simulink library "aerolibgravity2"  (R2020a)
settings: Solver=ode45  StartTime=0.0  StopTime=10.0  RelTol=1e-3
PostLoadFcn:
  | load_system('aerolibv1')
  | setsysloc('aerolibv1')
undefined symbols (not defined in the file or in its folder): aeroassertmsg, C, geoidgrid, ghCurrent, GM, latbp, lonbp, minYearCurrent, Newton, nMax10, nMax13, nMaxBetween, nMaxCurrent, R, Raphson, S, svCurrent, tabNMax10, tabNMax13, tabNMaxBetween
libraries: simulink x17, aerolibgravitysys x4
(part 2 of 4)

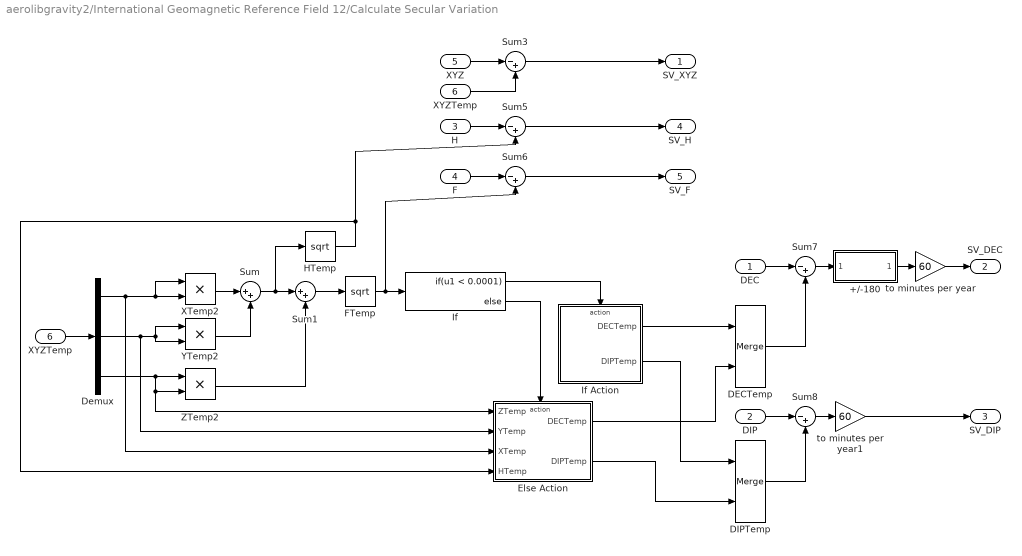
== system aerolibgravity2/International Geomagnetic Reference Field 12/Calculate Secular Variation ==
  DEC : Inport
  DIP : Inport  Port=2
  H : Inport  Port=3
  F : Inport  Port=4
  XYZ : Inport  Port=5
  XYZTemp : Inport  Port=6
  +/-180 : Subsystem
  DECTemp : Merge
  DIPTemp : Merge
  Demux : Demux  Outputs=3
  Else Action : Subsystem  TreatAsAtomicUnit=on
  FTemp : Sqrt  SaturateOnIntegerOverflow=on
  HTemp : Sqrt  SaturateOnIntegerOverflow=on
  If : If  IfExpression=u1 < 0.0001
  If Action : Subsystem  TreatAsAtomicUnit=on
  Sum : Sum  Inputs=|++
  Sum1 : Sum  Inputs=|++
  Sum{3,5..8} (5 alike) : Sum  Inputs=|-+
  XTemp2 : Product  RndMeth=Zero
  "XYZTemp " : InportShadow  Port=6
  YTemp2 : Product  RndMeth=Zero
  ZTemp2 : Product  RndMeth=Zero
  to minutes per year : Gain  Gain=60
  to minutes per year1 : Gain  Gain=60
  SV_XYZ : Outport  VectorParamsAs1DForOutWhenUnconnected=off
  SV_DEC : Outport  Port=2  VectorParamsAs1DForOutWhenUnconnected=off
  SV_DIP : Outport  Port=3  VectorParamsAs1DForOutWhenUnconnected=off
  SV_H : Outport  Port=4  VectorParamsAs1DForOutWhenUnconnected=off
  SV_F : Outport  Port=5  VectorParamsAs1DForOutWhenUnconnected=off
  wires:
  Sum3/1 -> SV_XYZ/1
  Demux/3 -> ZTemp2/1, ZTemp2/2, Else Action/1(ZTemp)
  Demux/2 -> YTemp2/2, YTemp2/1, Else Action/2(YTemp)
  Demux/1 -> XTemp2/2, XTemp2/1, Else Action/3(XTemp)
  XTemp2/1 -> Sum/1
  YTemp2/1 -> Sum/2
  Sum/1 -> Sum1/1, HTemp/1
  ZTemp2/1 -> Sum1/2
  Sum1/1 -> FTemp/1
  If/1 -> If Action/Action
  FTemp/1 -> If/1, Sum6/2
  If/2 -> Else Action/Action
  XYZ/1 -> Sum3/1
  HTemp/1 -> Else Action/4(HTemp), Sum5/2
  H/1 -> Sum5/1
  Sum5/1 -> SV_H/1
  F/1 -> Sum6/1
  Sum6/1 -> SV_F/1
  If Action/1(DECTemp) -> DECTemp/1
  Else Action/1(DECTemp) -> DECTemp/2
  DEC/1 -> Sum7/1
  DECTemp/1 -> Sum7/2
  If Action/2(DIPTemp) -> DIPTemp/1
  Else Action/2(DIPTemp) -> DIPTemp/2
  DIP/1 -> Sum8/1
  DIPTemp/1 -> Sum8/2
  Sum7/1 -> +/-180/1("DDEC ")
  Sum8/1 -> to minutes per year1/1
  to minutes per year/1 -> SV_DEC/1
  to minutes per year1/1 -> SV_DIP/1
  +/-180/1(DDEC) -> to minutes per year/1
  XYZTemp/1 -> Demux/1
  "XYZTemp "/1 -> Sum3/2

== system aerolibgravity2/International Geomagnetic Reference Field 12/Extrapolate or Interpolate ==
  dyear : Inport
  Extrapolation : Subsystem  TreatAsAtomicUnit=on
  If : If  IfExpression=u1 < 2015
  Interpolate : Subsystem  TreatAsAtomicUnit=on
  dyear1 : InportShadow
  dyear2 : InportShadow
  "gha " : Merge
  "ghb " : Merge
  "nMax " : Merge
  nMax : Outport  VectorParamsAs1DForOutWhenUnconnected=off
  gha : Outport  Port=2  VectorParamsAs1DForOutWhenUnconnected=off
  ghb : Outport  Port=3  VectorParamsAs1DForOutWhenUnconnected=off
  wires:
  If/1 -> Interpolate/Action
  If/2 -> Extrapolation/Action
  Interpolate/1(gha) -> "gha "/1
  Extrapolation/1(gha) -> "gha "/2
  Interpolate/2(ghb) -> "ghb "/1
  Extrapolation/2(ghb) -> "ghb "/2
  "gha "/1 -> gha/1
  "ghb "/1 -> ghb/1
  "nMax "/1 -> nMax/1
  Extrapolation/3(nMax) -> "nMax "/2
  Interpolate/3(nMax) -> "nMax "/1
  dyear/1 -> If/1
  dyear1/1 -> Extrapolation/1(dyear)
  dyear2/1 -> Interpolate/1(dyear)

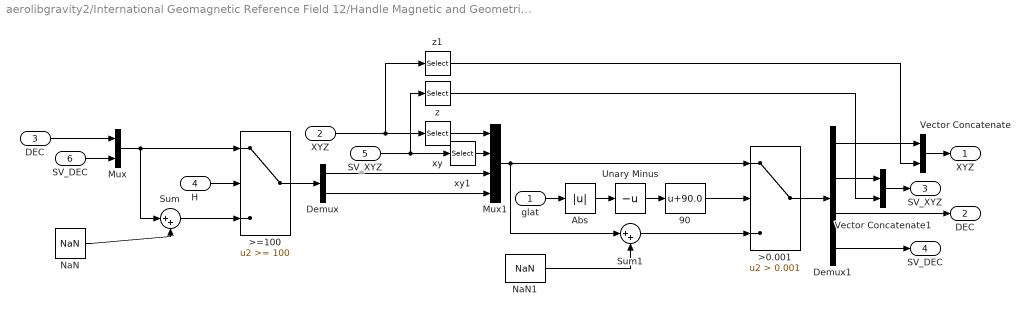
== system aerolibgravity2/International Geomagnetic Reference Field 12/Handle Magnetic and Geometric Poles ==
  glat : Inport
  "XYZ " : Inport  Port=2
  "DEC " : Inport  Port=3
  H : Inport  Port=4
  "SV_XYZ " : Inport  Port=5
  "SV_DEC " : Inport  Port=6
  90 : Bias  Bias=90.0
  >0.001 : Switch  Criteria=u2 > Threshold  Threshold=0.001
  >=100 : Switch  Threshold=100
  Abs : Abs
  Demux : Demux  Outputs=2
  Demux1 : Demux  Outputs=[2 2 1 1]
  Mux : Mux  Inputs=2
  Mux1 : Mux
  NaN : Constant  Value=NaN
  NaN1 : Constant  Value=NaN
  Sum : Sum  Inputs=|++
  Sum1 : Sum  Inputs=|++
  Unary Minus : UnaryMinus
  Vector Concatenate : Concatenate
  Vector Concatenate1 : Concatenate
  xy : Selector  InputPortWidth=3  IndexOptions=Index vector (dialog)  Indices=[1 2]  OutputSizes=1
  xy1 : Selector  InputPortWidth=3  IndexOptions=Index vector (dialog)  Indices=[1 2]  OutputSizes=1
  z : Selector  InputPortWidth=3  IndexOptions=Index vector (dialog)  Indices=3  OutputSizes=1
  z1 : Selector  InputPortWidth=3  IndexOptions=Index vector (dialog)  Indices=3  OutputSizes=1
  XYZ : Outport  Unit=nT  VectorParamsAs1DForOutWhenUnconnected=off
  DEC : Outport  Port=2  VectorParamsAs1DForOutWhenUnconnected=off
  SV_XYZ : Outport  Port=3  VectorParamsAs1DForOutWhenUnconnected=off
  SV_DEC : Outport  Port=4  VectorParamsAs1DForOutWhenUnconnected=off
  wires:
  z/1 -> Vector Concatenate1/2
  Vector Concatenate1/1 -> SV_XYZ/1
  z1/1 -> Vector Concatenate/2
  Vector Concatenate/1 -> XYZ/1
  xy1/1 -> Mux1/2
  xy/1 -> Mux1/1
  "XYZ "/1 -> z1/1, xy/1
  "SV_XYZ "/1 -> z/1, xy1/1
  H/1 -> >=100/2
  "DEC "/1 -> Mux/1
  "SV_DEC "/1 -> Mux/2
  Mux/1 -> >=100/1, Sum/1
  Sum/1 -> >=100/3
  NaN/1 -> Sum/2
  >=100/1 -> Demux/1
  Demux/1 -> Mux1/3
  Demux/2 -> Mux1/4
  glat/1 -> Abs/1
  Mux1/1 -> >0.001/1, Sum1/1
  >0.001/1 -> Demux1/1
  Demux1/1 -> Vector Concatenate/1
  Demux1/2 -> Vector Concatenate1/1
  Abs/1 -> Unary Minus/1
  Unary Minus/1 -> 90/1
  90/1 -> >0.001/2
  Demux1/3 -> DEC/1
  Demux1/4 -> SV_DEC/1
  NaN1/1 -> Sum1/2
  Sum1/1 -> >0.001/3

== system aerolibgravity2/International Geomagnetic Reference Field 12/Is decimal year within model limits ==
  u : Inport
  Assertion : Assertion  Enabled=off  AssertionFailFcn=evalin('base',callback)  StopWhenAssertionFail=off
  conjunction : Logic
  max_relop : RelationalOperator  Operator=<=  RndMeth=Nearest  InputSameDT=on
  max_val : Constant  Value=max  OutDataTypeStr=Inherit: Inherit via back propagation
  maxtype : DataTypeConversion  SaturateOnIntegerOverflow=on  RndMeth=Zero
  min_relop : RelationalOperator  Operator=<=  RndMeth=Nearest  InputSameDT=on
  min_val : Constant  Value=min  OutDataTypeStr=Inherit: Inherit via back propagation
  mintype : DataTypeConversion  SaturateOnIntegerOverflow=on  RndMeth=Zero
  out : Terminator
  wires:
  maxtype/1 -> max_relop/2
  mintype/1 -> min_relop/1
  conjunction/1 -> Assertion/1, out/1
  max_relop/1 -> conjunction/2
  min_relop/1 -> conjunction/1
  max_val/1 -> maxtype/1
  min_val/1 -> mintype/1
  u/1 -> max_relop/1, min_relop/2

== system aerolibgravity2/International Geomagnetic Reference Field 12/Length Conversion ==
  in : Inport
  Unit Conversion : UnitConversion
  out : Outport  Unit=m  VectorParamsAs1DForOutWhenUnconnected=off
  wires:
  in/1 -> Unit Conversion/1
  Unit Conversion/1 -> out/1

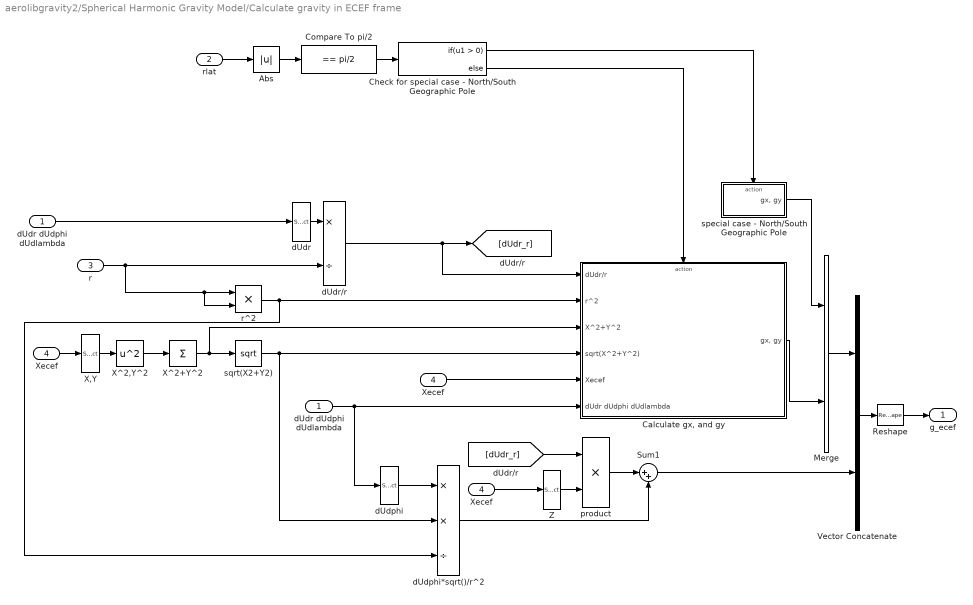
== system aerolibgravity2/Spherical Harmonic Gravity Model/Calculate gravity in ECEF frame ==
  dUdr dUdphi dUdlambda : Inport
  rlat : Inport  Port=2
  r : Inport  Port=3
  Xecef : Inport  Port=4
  " Xecef" : InportShadow  Port=4
  " Xecef " : InportShadow  Port=4
  " dUdphi " : Selector  InputPortWidth=3  IndexOptions=Index vector (dialog)  Indices=2  OutputSizes=1
  Abs : Abs
  "Calculate gx, and gy" : Subsystem
  Check for special case - North/South Geographic Pole : If
  Compare To pi/2 : simulink/Logic and Bit Operations/Compare To Constant  relop===  const=pi/2  OutDataTypeStr=uint8
  Merge : Merge
  Reshape : Reshape  OutputDimensionality=Row vector (2-D)
  Sum1 : Sum  Inputs=|++
  Vector Concatenate : Concatenate
  X,Y : Selector  InputPortWidth=3  IndexOptions=Index vector (dialog)  Indices=[1 2]  OutputSizes=1
  X^2+Y^2 : Sum  Inputs=+
  X^2,Y^2 : Math  Operator=square  SignedPower=on  SaturateOnIntegerOverflow=on
  "Z " : Selector  InputPortWidth=3  IndexOptions=Index vector (dialog)  Indices=3  OutputSizes=1
  dUdphi*sqrt()/r^2 : Product  Inputs=**/
  dUdr : Selector  InputPortWidth=3  IndexOptions=Index vector (dialog)  Indices=1  OutputSizes=1
  "dUdr dUdphi dUdlambda " : InportShadow
  dUdr/r : Product  Inputs=*/
  product : Product  RndMeth=Zero
  r^2 : Product  RndMeth=Zero
  special case - North/South Geographic Pole : Subsystem  TreatAsAtomicUnit=on
  sqrt(X2+Y2) : Sqrt  AlgorithmType=Newton-Raphson  SaturateOnIntegerOverflow=on
  g_ecef : Outport  VectorParamsAs1DForOutWhenUnconnected=off
  wires:
  rlat/1 -> Abs/1
  Merge/1 -> Vector Concatenate/1
  special case - North/South Geographic Pole/1("gx, gy") -> Merge/1
  Check for special case - North/South Geographic Pole/2 -> "Calculate gx, and gy"/Action
  "dUdr dUdphi dUdlambda "/1 -> " dUdphi "/1, "Calculate gx, and gy"/6("dUdr dUdphi dUdlambda ")
  " Xecef "/1 -> "Calculate gx, and gy"/5(" Xecef")
  Abs/1 -> Compare To pi/2/1
  Compare To pi/2/1 -> Check for special case - North/South Geographic Pole/1
  Check for special case - North/South Geographic Pole/1 -> special case - North/South Geographic Pole/Action
  Vector Concatenate/1 -> Reshape/1
  "Calculate gx, and gy"/1("gx, gy") -> Merge/2
  Sum1/1 -> Vector Concatenate/2
  " Xecef"/1 -> "Z "/1
  product/1 -> Sum1/1
  "Z "/1 -> product/2
  [dUdr_r] -> product/1
  dUdphi*sqrt()/r^2/1 -> Sum1/2
  " dUdphi "/1 -> dUdphi*sqrt()/r^2/1
  r^2/1 -> "Calculate gx, and gy"/2(r^2), dUdphi*sqrt()/r^2/3
  sqrt(X2+Y2)/1 -> dUdphi*sqrt()/r^2/2, "Calculate gx, and gy"/4(sqrt(X^2+Y^2))
  dUdr/r/1 -> "Calculate gx, and gy"/1(dUdr/r), [dUdr_r]
  X^2+Y^2/1 -> sqrt(X2+Y2)/1, "Calculate gx, and gy"/3(X^2+Y^2)
  X^2,Y^2/1 -> X^2+Y^2/1
  X,Y/1 -> X^2,Y^2/1
  dUdr/1 -> dUdr/r/1
  Reshape/1 -> g_ecef/1
  r/1 -> r^2/1, r^2/2, dUdr/r/2
  dUdr dUdphi dUdlambda/1 -> dUdr/1
  Xecef/1 -> X,Y/1

== system aerolibgravity2/Spherical Harmonic Gravity Model/Compute gravity in spherical coordinates ==
  srlon_array : Inport
  crlon_array : Inport  Port=2
  trlat : Inport  Port=3
  srphi : Inport  Port=4
  crphi : Inport  Port=5
  r : Inport  Port=6
  Compute normalized associated legendre polynomials and gravity : S-Function  FunctionName=saeroshgravity  Parameters=GM, R, C, S, int16(degree)  SFunctionDeploymentMode=off  EnableBusSupport=off
  Vector Concatenate1 : Concatenate  NumInputs=3
  dUdr dUdphi dUdlambda : Outport  VectorParamsAs1DForOutWhenUnconnected=off
  wires:
  crphi/1 -> Compute normalized associated legendre polynomials and gravity/5
  Vector Concatenate1/1 -> dUdr dUdphi dUdlambda/1
  Compute normalized associated legendre polynomials and gravity/3 -> Vector Concatenate1/3
  Compute normalized associated legendre polynomials and gravity/2 -> Vector Concatenate1/2
  Compute normalized associated legendre polynomials and gravity/1 -> Vector Concatenate1/1
  trlat/1 -> Compute normalized associated legendre polynomials and gravity/1
  srlon_array/1 -> Compute normalized associated legendre polynomials and gravity/2  "srlon"
  crlon_array/1 -> Compute normalized associated legendre polynomials and gravity/3  "crlon"
  srphi/1 -> Compute normalized associated legendre polynomials and gravity/4
  r/1 -> Compute normalized associated legendre polynomials and gravity/6

== system aerolibgravity2/Spherical Harmonic Gravity Model/Find radius, geocentric latitude, and longitude ==
  Xecef : Inport
  Divide : Product  Inputs=*/
  Dot Product : DotProduct  InputSameDT=on  OutDataTypeStr=Inherit: Inherit via internal rule
  Sum of Elements : Sum  Inputs=+
  X : Selector  InputPortWidth=3  IndexOptions=Index vector (dialog)  Indices=1  OutputSizes=1
  Y : Selector  InputPortWidth=3  IndexOptions=Index vector (dialog)  Indices=2  OutputSizes=1
  Z : Selector  InputPortWidth=3  IndexOptions=Index vector (dialog)  Indices=3  OutputSizes=1
  "r " : Sqrt  AlgorithmType=Newton-Raphson  SaturateOnIntegerOverflow=on
  "rlat " : Trigonometry  Operator=asin
  "rlon " : Trigonometry  Operator=atan2
  rlon : Outport  VectorParamsAs1DForOutWhenUnconnected=off
  rlat : Outport  Port=2  VectorParamsAs1DForOutWhenUnconnected=off
  r : Outport  Port=3  VectorParamsAs1DForOutWhenUnconnected=off
  wires:
  Y/1 -> "rlon "/1
  X/1 -> "rlon "/2
  "rlon "/1 -> rlon/1
  "rlat "/1 -> rlat/1
  Z/1 -> Divide/1
  Divide/1 -> "rlat "/1
  "r "/1 -> r/1, Divide/2
  Sum of Elements/1 -> "r "/1
  Dot Product/1 -> Sum of Elements/1
  Xecef/1 -> X/1, Y/1, Dot Product/2, Dot Product/1, Z/1

== system aerolibgravity2/Spherical Harmonic Gravity Model/Get Cosine and Sine of Latitude and Longitude ==
  rlon : Inport
  rlat : Inport  Port=2
  Constant : Constant  Value=pi/2
  Demux : Demux  Outputs=2
      settings: DisplayOption=none
  Demux1 : Demux  Outputs=2
      settings: DisplayOption=none
  Mux : Mux  Inputs=2
  Sum : Sum  Inputs=|-+
  Test for less than eps : Subsystem
  "Test for less than eps " : Subsystem
  sincos : Trigonometry  Operator=sincos
  sincos1 : Trigonometry  Operator=tan
  srlon : Outport  VectorParamsAs1DForOutWhenUnconnected=off
  crlon : Outport  Port=2  VectorParamsAs1DForOutWhenUnconnected=off
  trlat : Outport  Port=3  VectorParamsAs1DForOutWhenUnconnected=off
  srphi : Outport  Port=4  VectorParamsAs1DForOutWhenUnconnected=off
  crphi : Outport  Port=5  VectorParamsAs1DForOutWhenUnconnected=off
  wires:
  "Test for less than eps "/1(Out1) -> crphi/1
  Test for less than eps/1(Out1) -> srphi/1
  sincos1/1 -> trlat/1
  Constant/1 -> Sum/2
  Sum/1 -> Mux/2
  Mux/1 -> sincos/1
  sincos/1 -> Demux/1
  sincos/2 -> Demux1/1
  rlon/1 -> Mux/1
  rlat/1 -> Sum/1, sincos1/1
  Demux/1 -> srlon/1
  Demux1/1 -> crlon/1
  Demux/2 -> Test for less than eps/1(In1)
  Demux1/2 -> "Test for less than eps "/1(In1)

== system aerolibgravity2/Spherical Harmonic Gravity Model/sin(m_lon) & cos(m_lon) ==
  srlon : Inport
  crlon : Inport  Port=2
  For Iterator Subsystem : Subsystem  TreatAsAtomicUnit=on
  Test for less than eps : Subsystem
  "Test for less than eps " : Subsystem
  srlon_array : Outport  InitialOutput=[ zeros(1,degree+1) ]  VectorParamsAs1DForOutWhenUnconnected=off
  crlon_array : Outport  Port=2  InitialOutput=[ zeros(1,degree+1) ]  VectorParamsAs1DForOutWhenUnconnected=off
  wires:
  "Test for less than eps "/1(Out1) -> For Iterator Subsystem/2(crlon[1])
  srlon/1 -> Test for less than eps/1(In1)
  crlon/1 -> "Test for less than eps "/1(In1)
  For Iterator Subsystem/1(srlon_array) -> srlon_array/1
  For Iterator Subsystem/2(crlon_array) -> crlon_array/1
  Test for less than eps/1(Out1) -> For Iterator Subsystem/1(srlon[1])

== system aerolibgravity2/World Magnetic Model/Is time within model limits ==
  u : Inport
  Assertion : Assertion  AssertionFailFcn=evalin('base',callback)
  conjunction : Logic
  max_relop : RelationalOperator  Operator=<=  RndMeth=Nearest  InputSameDT=on
  max_val : Constant  Value=max
  maxtype : DataTypeConversion  SaturateOnIntegerOverflow=on  RndMeth=Zero
  min_relop : RelationalOperator  Operator=<=  RndMeth=Nearest  InputSameDT=on
  min_val : Constant  Value=min
  mintype : DataTypeConversion  SaturateOnIntegerOverflow=on  RndMeth=Zero
  out : Terminator
  wires:
  maxtype/1 -> max_relop/2
  mintype/1 -> min_relop/1
  conjunction/1 -> Assertion/1, out/1
  max_relop/1 -> conjunction/2
  min_relop/1 -> conjunction/1
  max_val/1 -> maxtype/1
  min_val/1 -> mintype/1
  u/1 -> max_relop/1, min_relop/2

== system aerolibgravity2/World Magnetic Model/Length Conversion ==
  in : Inport
  Unit Conversion : UnitConversion
  out : Outport  Unit=m  VectorParamsAs1DForOutWhenUnconnected=off
  wires:
  in/1 -> Unit Conversion/1
  Unit Conversion/1 -> out/1

== system aerolibgravity2/World Magnetic Model/MagField Conversion ==
  in : Inport  Unit=nT
  Unit Conversion : UnitConversion
  out : Outport  Unit=nT  VectorParamsAs1DForOutWhenUnconnected=off
  wires:
  in/1 -> Unit Conversion/1
  Unit Conversion/1 -> out/1

== system aerolibgravity2/World Magnetic Model/MagField Conversion1 ==
  in : Inport  Unit=nT
  Unit Conversion : UnitConversion
  out : Outport  Unit=nT  VectorParamsAs1DForOutWhenUnconnected=off
  wires:
  in/1 -> Unit Conversion/1
  Unit Conversion/1 -> out/1

== system aerolibgravity2/Zonal Harmonic Gravity Model/Calculate gravity in ECEF frame ==
  g_radial : Inport
  g_trans : Inport  Port=2
  r : Inport  Port=3
  Xecef : Inport  Port=4
  Divide : Product  Inputs=*/
  Mux : Mux  Inputs=3
  Reshape : Reshape  OutputDimensionality=Row vector (2-D)
  gx & gy : Subsystem
  gz : Subsystem
  g_ecef : Outport  VectorParamsAs1DForOutWhenUnconnected=off
  wires:
  Reshape/1 -> g_ecef/1
  gz/1(gz) -> Mux/3
  gx & gy/2(gy) -> Mux/2
  gx & gy/1(gx) -> Mux/1
  Mux/1 -> Reshape/1
  g_trans/1 -> gx & gy/2(g_trans), gz/3(g_trans)
  Divide/1 -> gx & gy/4(g_radial/r), gz/1(g_radial/r)
  r/1 -> gx & gy/3(r), gz/2(r), Divide/2
  g_radial/1 -> Divide/1
  Xecef/1 -> gz/4(Xecef), gx & gy/1(Xecef)

== system aerolibgravity2/Zonal Harmonic Gravity Model/Find radius and geocentric latitude ==
  Xecef : Inport
  Divide : Product  Inputs=*/
  Dot Product : DotProduct  InputSameDT=on  OutDataTypeStr=Inherit: Inherit via internal rule
  Selector : Selector  InputPortWidth=3  IndexOptions=Index vector (dialog)  Indices=3  OutputSizes=1
  Sum of Elements : Sum  Inputs=+
  "rlat " : Trigonometry  Operator=asin
  sqrt : Sqrt  AlgorithmType=Newton-Raphson  SaturateOnIntegerOverflow=on
  rlat : Outport  VectorParamsAs1DForOutWhenUnconnected=off
  r : Outport  Port=2  VectorParamsAs1DForOutWhenUnconnected=off
  wires:
  "rlat "/1 -> rlat/1
  Selector/1 -> Divide/1
  Divide/1 -> "rlat "/1
  sqrt/1 -> r/1, Divide/2
  Sum of Elements/1 -> sqrt/1
  Dot Product/1 -> Sum of Elements/1
  Xecef/1 -> Dot Product/1, Dot Product/2, Selector/1

== system aerolibgravity2/Geoid Height/Format Output/Change Units ==
  in : Inport  Unit=m
  Unit Conversion : UnitConversion
  out : Outport  Unit=m  VectorParamsAs1DForOutWhenUnconnected=off
  wires:
  in/1 -> Unit Conversion/1
  Unit Conversion/1 -> out/1

== system aerolibgravity2/Geoid Height/Format Output/Truncate ==
  In1 : Inport
  Constant1 : Constant  Value=100  OutDataTypeStr=double
  Divide : Product  Inputs=*/
  Product : Product  RndMeth=Zero
  Rounding Function : Rounding  Operator=fix
  Out1 : Outport  VectorParamsAs1DForOutWhenUnconnected=off
  wires:
  Divide/1 -> Out1/1
  In1/1 -> Product/1
  Constant1/1 -> Divide/2, Product/2
  Rounding Function/1 -> Divide/1
  Product/1 -> Rounding Function/1

== system aerolibgravity2/Geoid Height/Format Output/Truncate1 ==
  In1 : Inport
  Constant1 : Constant  Value=100  OutDataTypeStr=double
  Divide : Product  Inputs=*/
  Product : Product  RndMeth=Zero
  Rounding Function : Rounding  Operator=fix
  Out1 : Outport  VectorParamsAs1DForOutWhenUnconnected=off
  wires:
  Product/1 -> Rounding Function/1
  Rounding Function/1 -> Divide/1
  Constant1/1 -> Product/2, Divide/2
  In1/1 -> Product/1
  Divide/1 -> Out1/1

== system aerolibgravity2/Geoid Height/Wrap Latitude/If Action Subsystem ==
  Lat : Inport
  Lon : Inport  Port=2
  Action Port : ActionPort  PropagateVarSize=During execution
  Abs : Abs
  Add : Sum
  Add1 : Sum  Inputs=-+
  Add2 : Sum  Inputs=+-
  Constant1 : Constant  Value=double(90)
  Constant2 : Constant  Value=double(180)
  Divide : Product  Inputs=**
  Sign : Signum
  Lat1 : Outport  VectorParamsAs1DForOutWhenUnconnected=off
  Lon1 : Outport  Port=2  VectorParamsAs1DForOutWhenUnconnected=off
  wires:
  Lon/1 -> Add/1
  Constant2/1 -> Add/2
  Add/1 -> Lon1/1
  Divide/1 -> Lat1/1
  Abs/1 -> Add2/1
  Add2/1 -> Add1/1
  Constant1/1 -> Add2/2, Add1/2
  Sign/1 -> Divide/1
  Add1/1 -> Divide/2
  Lat/1 -> Abs/1, Sign/1

== system aerolibgravity2/Geoid Height/Wrap Latitude/If Action Subsystem1 ==
  Lat : Inport
  Lon : Inport  Port=2
  Action Port : ActionPort  PropagateVarSize=During execution
  Lat1 : Outport  VectorParamsAs1DForOutWhenUnconnected=off
  Lon1 : Outport  Port=2  VectorParamsAs1DForOutWhenUnconnected=off
  wires:
  Lat/1 -> Lat1/1
  Lon/1 -> Lon1/1

== system aerolibgravity2/Geoid Height/Wrap Latitude/Wrap Latitude 180 ==
  lat : Inport
  Constant : Constant  Value=double(360)
  Constant1 : Constant  Value=double(180)
  Math Function : Math  Operator=mod  SignedPower=on  SaturateOnIntegerOverflow=on
  Sum : Sum  Inputs=++|
  Sum1 : Sum  Inputs=-+|
  lat 180 : Outport  VectorParamsAs1DForOutWhenUnconnected=off
  wires:
  lat/1 -> Sum/2
  Sum/1 -> Math Function/1
  Constant/1 -> Math Function/2
  Math Function/1 -> Sum1/2
  Sum1/1 -> lat 180/1
  Constant1/1 -> Sum/1, Sum1/1

== system aerolibgravity2/Geoid Height/Wrap Longitude/If Action Subsystem ==
  Lon : Inport
  Action Port : ActionPort  PropagateVarSize=During execution
  Constant1 : Constant  Value=double(360)
  Math Function : Math  Operator=mod  SignedPower=on  SaturateOnIntegerOverflow=on
  Lon1 : Outport  VectorParamsAs1DForOutWhenUnconnected=off
  wires:
  Constant1/1 -> Math Function/2
  Lon/1 -> Math Function/1
  Math Function/1 -> Lon1/1

== system aerolibgravity2/Geoid Height/Wrap Longitude/If Action Subsystem1 ==
  Lon : Inport
  Action Port : ActionPort  PropagateVarSize=During execution
  Lon1 : Outport  VectorParamsAs1DForOutWhenUnconnected=off
  wires:
  Lon/1 -> Lon1/1

== system aerolibgravity2/International Geomagnetic Reference Field 12/Calculate Field/Compute magnetic vector in spherical coordinates ==
  gha : Inport
  ghb : Inport  Port=2
  r : Inport  Port=3
  clat : Inport  Port=4
  slat : Inport  Port=5
  sd : Inport  Port=6
  cd : Inport  Port=7
  crlon : Inport  Port=8
  srlon : Inport  Port=9
  nMax : Inport  Port=10
  Enable : EnablePort  PropagateVarSize=During execution
  "Calculate X, Z, XTemp and ZTemp" : Subsystem
  Compute magnetic vector in spherical coordinates : Subsystem  TreatAsAtomicUnit=on
  Constant2 : Constant  Value=0.5  OutDataTypeStr=Inherit: Inherit via back propagation
  Product3 : Product  Inputs=***  SaturateOnIntegerOverflow=on  OutDataTypeStr=Inherit: Same as first input
  aor : Product  Inputs=*/  SaturateOnIntegerOverflow=on  OutDataTypeStr=Inherit: Same as first input
  nMax+3 : Bias  Bias=3.0
  re : Constant  Value=6371.2  OutDataTypeStr=Inherit: Inherit via back propagation
  XYZ : Outport  InitialOutput=[0 0 0]  VectorParamsAs1DForOutWhenUnconnected=off
  XYZTemp : Outport  Port=2  InitialOutput=[0 0 0]  VectorParamsAs1DForOutWhenUnconnected=off
  wires:
  Product3/1 -> Compute magnetic vector in spherical coordinates/8(cntMax)
  Constant2/1 -> Product3/3
  nMax+3/1 -> Product3/2
  nMax/1 -> Product3/1, nMax+3/1
  gha/1 -> Compute magnetic vector in spherical coordinates/1(gha)
  ghb/1 -> Compute magnetic vector in spherical coordinates/2(ghb)
  re/1 -> aor/1
  aor/1 -> Compute magnetic vector in spherical coordinates/3(aor)
  Compute magnetic vector in spherical coordinates/1(XYZ) -> "Calculate X, Z, XTemp and ZTemp"/1("XYZ ")
  Compute magnetic vector in spherical coordinates/2(XYZTemp) -> "Calculate X, Z, XTemp and ZTemp"/2("XYZTemp ")
  "Calculate X, Z, XTemp and ZTemp"/1(XYZ) -> XYZ/1
  "Calculate X, Z, XTemp and ZTemp"/2(XYZTemp) -> XYZTemp/1
  r/1 -> aor/2
  clat/1 -> Compute magnetic vector in spherical coordinates/4(clat)
  slat/1 -> Compute magnetic vector in spherical coordinates/5(slat)
  crlon/1 -> Compute magnetic vector in spherical coordinates/6(crlon)
  srlon/1 -> Compute magnetic vector in spherical coordinates/7(srlon)
  sd/1 -> "Calculate X, Z, XTemp and ZTemp"/3(sd)
  cd/1 -> "Calculate X, Z, XTemp and ZTemp"/4(cd)

== system aerolibgravity2/International Geomagnetic Reference Field 12/Calculate Field/Convert from geodetic to spherical coordinates ==
  alt : Inport
  srlat : Inport  Port=2
  srlat2 : Inport  Port=3
  crlat2 : Inport  Port=4
  crlat : Inport  Port=5
  Enable : EnablePort  PropagateVarSize=During execution
  Demux : Demux
      settings: DisplayOption=none
  Demux1 : Demux
      settings: DisplayOption=none
  Demux3 : Demux  Outputs=2
      settings: DisplayOption=none
  Mux : Mux
  Selector : Selector  InputPortWidth=4  IndexOptions=Index vector (dialog)  Indices=[1 2]  OutputSizes=1
  a2 : Constant  Value=40680631.59  OutDataTypeStr=Inherit: Inherit via back propagation
  "alt " : InportShadow
  b2 : Constant  Value=40408299.98  OutDataTypeStr=Inherit: Inherit via back propagation
  calculate cd : Subsystem
  calculate clat & slat : Subsystem
  calculate d : Subsystem
  calculate r2 : Subsystem
  calculate sd : Subsystem
  r : Outport  InitialOutput=[40680631]  VectorParamsAs1DForOutWhenUnconnected=off
  clat : Outport  Port=2  InitialOutput=[0]  VectorParamsAs1DForOutWhenUnconnected=off
  slat : Outport  Port=3  InitialOutput=[1]  VectorParamsAs1DForOutWhenUnconnected=off
  sd : Outport  Port=4  InitialOutput=[0]  VectorParamsAs1DForOutWhenUnconnected=off
  cd : Outport  Port=5  InitialOutput=[0]  VectorParamsAs1DForOutWhenUnconnected=off
  wires:
  Demux/3 -> calculate d/3(srlat2)
  Selector/1 -> Demux3/1
  Demux3/2 -> calculate sd/3(b2)
  Demux3/1 -> calculate sd/2(a2)
  Mux/1 -> Demux/1, Demux1/1, Selector/1
  Demux1/3 -> calculate r2/4(srlat2)
  Demux1/2 -> calculate r2/3(b2)
  Demux1/1 -> calculate r2/2(a2)
  Demux/1 -> calculate d/1(a2)
  Demux/2 -> calculate d/2(b2)
  b2/1 -> Mux/2
  a2/1 -> Mux/1
  calculate sd/1(sd) -> calculate clat & slat/1(sd), sd/1
  crlat/1 -> calculate sd/5(crlat), calculate clat & slat/3(crlat)
  calculate cd/1(cd) -> cd/1, calculate clat & slat/4(cd)
  calculate d/2(d) -> calculate sd/1(d), calculate cd/3(d), calculate r2/7(d)
  calculate r2/1(r) -> calculate cd/2(r), calculate sd/4(r), r/1
  calculate clat & slat/2(slat) -> slat/1  "slat"
  calculate clat & slat/1(clat) -> clat/1  "clat"
  srlat/1 -> calculate sd/6(srlat), calculate clat & slat/2(srlat)
  crlat2/1 -> Mux/4
  alt/1 -> calculate r2/1(alt)
  srlat2/1 -> Mux/3
  Demux/4 -> calculate d/4(crlat2)
  Demux1/4 -> calculate r2/5(crlat2)
  calculate d/1(c2) -> calculate r2/6(c2)
  "alt "/1 -> calculate cd/1(alt)

== system aerolibgravity2/International Geomagnetic Reference Field 12/Calculate Field/Get Cosine and Sine of Latitude and Longitude ==
  lon : Inport  Unit=deg
  lat : Inport  Port=2  Unit=deg
  Enable : EnablePort  PropagateVarSize=During execution
  300 ft from North & South poles : Subsystem
  Angle Conversion : Subsystem
  Demux : Demux  Outputs=2
      settings: DisplayOption=none
  Demux1 : Demux  Outputs=2
      settings: DisplayOption=none
  Mux : Mux  Inputs=2
  Product : Product  OutDataTypeStr=Inherit: Inherit via back propagation  SaturateOnIntegerOverflow=on
  Product1 : Product  OutDataTypeStr=Inherit: Inherit via back propagation  SaturateOnIntegerOverflow=on
  sincos : Trigonometry  Operator=sincos
  srlat : Outport  InitialOutput=[0]  VectorParamsAs1DForOutWhenUnconnected=off
  srlat2 : Outport  Port=2  InitialOutput=[0]  VectorParamsAs1DForOutWhenUnconnected=off
  crlat2 : Outport  Port=3  InitialOutput=[0]  VectorParamsAs1DForOutWhenUnconnected=off
  crlat : Outport  Port=4  InitialOutput=[0]  VectorParamsAs1DForOutWhenUnconnected=off
  crlon : Outport  Port=5  InitialOutput=[1]  VectorParamsAs1DForOutWhenUnconnected=off
  srlon : Outport  Port=6  InitialOutput=[0]  VectorParamsAs1DForOutWhenUnconnected=off
  wires:
  Demux1/2 -> 300 ft from North & South poles/1("crlat ")
  Demux/2 -> Product/2, Product/1, srlat/1
  Product1/1 -> crlat2/1
  Product/1 -> srlat2/1
  Demux1/1 -> crlon/1  "crlon"
  Demux/1 -> srlon/1  "srlon"
  lat/1 -> Mux/2
  lon/1 -> Mux/1
  sincos/2 -> Demux1/1
  sincos/1 -> Demux/1
  Mux/1 -> Angle Conversion/1(in)
  Angle Conversion/1(out) -> sincos/1
  300 ft from North & South poles/1(crlat) -> Product1/2, Product1/1, crlat/1

== system aerolibgravity2/International Geomagnetic Reference Field 12/Calculate Field/Has altitude or latitude changed ==
  lat : Inport
  alt : Inport  Port=2
  Logical Operator : Logic  Operator=OR  AllPortsSameDT=off
  Relational Operator : RelationalOperator  Operator=~=  RndMeth=Nearest
  Relational Operator1 : RelationalOperator  Operator=~=  RndMeth=Nearest
  oalt : Memory  InitialCondition=-1000  InheritSampleTime=on
  olat : Memory  InitialCondition=-1000  InheritSampleTime=on
  Alt_Lat change : Outport  VectorParamsAs1DForOutWhenUnconnected=off
  wires:
  Logical Operator/1 -> Alt_Lat change/1
  lat/1 -> olat/1, Relational Operator/1
  Relational Operator1/1 -> Logical Operator/2
  Relational Operator/1 -> Logical Operator/1
  oalt/1 -> Relational Operator1/2
  olat/1 -> Relational Operator/2
  alt/1 -> oalt/1, Relational Operator1/1

== system aerolibgravity2/International Geomagnetic Reference Field 12/Calculate Field/Has longitude changed  ==
  lon : Inport
  Relational Operator : RelationalOperator  Operator=~=  RndMeth=Nearest
  olon : Memory  InitialCondition=-1000  InheritSampleTime=on
  Longitude change : Outport  VectorParamsAs1DForOutWhenUnconnected=off
  wires:
  Relational Operator/1 -> Longitude change/1
  lon/1 -> olon/1, Relational Operator/1
  olon/1 -> Relational Operator/2

== system aerolibgravity2/International Geomagnetic Reference Field 12/Calculate H, F, DEC,& DIP/Else Action ==
  Z : Inport
  Y : Inport  Port=2
  X : Inport  Port=3
  H : Inport  Port=4
  Action Port : ActionPort
  Angle Conversion : Subsystem
  "DEC " : Merge
  Else Action : Subsystem  TreatAsAtomicUnit=on
  If : If  IfExpression=u1 < 0.0001
  If Action : Subsystem  TreatAsAtomicUnit=on
  Trigonometric Function : Trigonometry  Operator=atan2
  DEC : Outport  InitialOutput=0  VectorParamsAs1DForOutWhenUnconnected=off
  DIP : Outport  Port=2  InitialOutput=0  VectorParamsAs1DForOutWhenUnconnected=off
  wires:
  If Action/1(DEC) -> "DEC "/1
  Else Action/1(DEC) -> "DEC "/2
  Y/1 -> Else Action/3(Y)
  X/1 -> Else Action/2(X)
  If/2 -> Else Action/Action
  If/1 -> If Action/Action
  Angle Conversion/1(out) -> DIP/1
  H/1 -> Else Action/1(H), If/1, Trigonometric Function/2
  Z/1 -> Trigonometric Function/1
  Trigonometric Function/1 -> Angle Conversion/1(in)
  "DEC "/1 -> DEC/1

== system aerolibgravity2/International Geomagnetic Reference Field 12/Calculate H, F, DEC,& DIP/If Action ==
  Action Port : ActionPort
  NaN : Constant  Value=NaN
  NaN1 : Constant  Value=NaN
  DEC : Outport  Unit=deg  InitialOutput=0  VectorParamsAs1DForOutWhenUnconnected=off
  DIP : Outport  Port=2  Unit=deg  InitialOutput=0  VectorParamsAs1DForOutWhenUnconnected=off
  wires:
  NaN/1 -> DEC/1
  NaN1/1 -> DIP/1

== system aerolibgravity2/International Geomagnetic Reference Field 12/Calculate Secular Variation/+//-180 ==
  "DDEC " : Inport
  +360 : Bias  Bias=360.0
  -360 : Bias  Bias=-360.0
  >-180 : Switch  Criteria=u2 > Threshold  Threshold=-180
  >180 : Switch  Criteria=u2 > Threshold  Threshold=180
  DDEC : Outport  VectorParamsAs1DForOutWhenUnconnected=off
  wires:
  "DDEC "/1 -> >180/3, >180/2, -360/1
  >180/1 -> >-180/1, >-180/2, +360/1
  >-180/1 -> DDEC/1
  +360/1 -> >-180/3
  -360/1 -> >180/1

== system aerolibgravity2/International Geomagnetic Reference Field 12/Calculate Secular Variation/Else Action ==
  ZTemp : Inport
  YTemp : Inport  Port=2
  XTemp : Inport  Port=3
  HTemp : Inport  Port=4
  Action Port : ActionPort
  Angle Conversion : Subsystem
  "DECTemp " : Merge
  Else Action : Subsystem  TreatAsAtomicUnit=on
  If : If  IfExpression=u1 < 0.0001
  If Action : Subsystem  TreatAsAtomicUnit=on
  Trigonometric Function : Trigonometry  Operator=atan2
  DECTemp : Outport  Unit=deg  InitialOutput=0  VectorParamsAs1DForOutWhenUnconnected=off
  DIPTemp : Outport  Port=2  Unit=deg  InitialOutput=0  VectorParamsAs1DForOutWhenUnconnected=off
  wires:
  "DECTemp "/1 -> DECTemp/1
  Trigonometric Function/1 -> Angle Conversion/1(in)
  ZTemp/1 -> Trigonometric Function/1
  HTemp/1 -> Trigonometric Function/2, If/1, Else Action/1(HTemp)
  Angle Conversion/1(out) -> DIPTemp/1
  If/1 -> If Action/Action
  If/2 -> Else Action/Action
  XTemp/1 -> Else Action/2(XTemp)
  YTemp/1 -> Else Action/3(YTemp)
  Else Action/1(DECTemp) -> "DECTemp "/2
  If Action/1(DECTemp) -> "DECTemp "/1

== system aerolibgravity2/International Geomagnetic Reference Field 12/Calculate Secular Variation/If Action ==
  Action Port : ActionPort
  NaN : Constant  Value=NaN
  NaN1 : Constant  Value=NaN
  DECTemp : Outport  Unit=deg  InitialOutput=0  VectorParamsAs1DForOutWhenUnconnected=off
  DIPTemp : Outport  Port=2  Unit=deg  InitialOutput=0  VectorParamsAs1DForOutWhenUnconnected=off
  wires:
  NaN/1 -> DECTemp/1
  NaN1/1 -> DIPTemp/1

== system aerolibgravity2/International Geomagnetic Reference Field 12/Extrapolate or Interpolate/Extrapolation ==
  dyear : Inport
  Action Port : ActionPort
  Bias : Bias  Bias=1.0
  Constant : Constant  Value=nMaxCurrent
  Product : Product  RndMeth=Zero
  Product1 : Product  RndMeth=Zero
  Sum : Sum  Inputs=|+-
  Sum1 : Sum  Inputs=|++
  Sum2 : Sum  Inputs=++|
  ghCurrent : Constant  Value=ghCurrent  VectorParams1D=off
  minYearCurrent : Constant  Value=minYearCurrent
  svCurrent : Constant  Value=svCurrent  VectorParams1D=off
  gha : Outport  InitialOutput=zeros(195,1)  VectorParamsAs1DForOutWhenUnconnected=off
  ghb : Outport  Port=2  InitialOutput=zeros(195,1)  VectorParamsAs1DForOutWhenUnconnected=off
  nMax : Outport  Port=3  InitialOutput=nMaxCurrent  VectorParamsAs1DForOutWhenUnconnected=off
  wires:
  minYearCurrent/1 -> Sum/2
  dyear/1 -> Sum/1
  Sum/1 -> Bias/1, Product/2
  Bias/1 -> Product1/1
  svCurrent/1 -> Product1/2, Product/1
  Product1/1 -> Sum1/1
  ghCurrent/1 -> Sum1/2, Sum2/1
  Product/1 -> Sum2/2
  Sum2/1 -> gha/1
  Sum1/1 -> ghb/1
  Constant/1 -> nMax/1

== system aerolibgravity2/International Geomagnetic Reference Field 12/Extrapolate or Interpolate/Interpolate ==
  dyear : Inport
  Action Port : ActionPort
  1900-1990 : Subsystem
  1990-1995 : Subsystem
  1995-2010 : Subsystem
  If : If  IfExpression=u1 < 1990.0  ElseIfExpressions=u1 >= 1995.0
  dyear1 : InportShadow
  dyear2 : InportShadow
  dyear3 : InportShadow
  "gha " : Merge  Inputs=3
  "ghb " : Merge  Inputs=3
  "nMax " : Merge  Inputs=3
  gha : Outport  VectorParamsAs1DForOutWhenUnconnected=off
  ghb : Outport  Port=2  VectorParamsAs1DForOutWhenUnconnected=off
  nMax : Outport  Port=3  VectorParamsAs1DForOutWhenUnconnected=off
  wires:
  dyear/1 -> If/1
  If/1 -> 1900-1990/Action
  If/3 -> 1990-1995/Action
  If/2 -> 1995-2010/Action
  dyear1/1 -> 1900-1990/1(dyear)
  dyear2/1 -> 1995-2010/1(dyear)
  dyear3/1 -> 1990-1995/1(dyear)
  1900-1990/1(gha) -> "gha "/1
  1995-2010/1(gha) -> "gha "/2
  1990-1995/1(gha) -> "gha "/3
  1990-1995/2(ghb) -> "ghb "/3
  1995-2010/2(ghb) -> "ghb "/2
  1900-1990/2(ghb) -> "ghb "/1
  "gha "/1 -> gha/1
  "ghb "/1 -> ghb/1
  "nMax "/1 -> nMax/1
  1900-1990/3(nMax) -> "nMax "/1
  1995-2010/3(nMax) -> "nMax "/2
  1990-1995/3(nMax) -> "nMax "/3

== system aerolibgravity2/Spherical Harmonic Gravity Model/Calculate gravity in ECEF frame/Calculate gx, and gy ==
  dUdr/r : Inport
  r^2 : Inport  Port=2
  X^2+Y^2 : Inport  Port=3
  sqrt(X^2+Y^2) : Inport  Port=4
  " Xecef" : Inport  Port=5
  "dUdr dUdphi dUdlambda " : Inport  Port=6
  Action Port : ActionPort
  " Xecef " : InportShadow  Port=5
  (r^2)*sqrt() : Product  RndMeth=Zero
  Gain : Gain  Gain=[-1 1]
  Product : Product  RndMeth=Zero
  Product1 : Product  RndMeth=Zero
  Sum : Sum  Inputs=|+-
  Sum2 : Sum  Inputs=++|
  "X,Y " : Selector  InputPortWidth=3  IndexOptions=Index vector (dialog)  Indices=[1 2]  OutputSizes=1
  Xecef : InportShadow  Port=5
  Y,X : Selector  InputPortWidth=3  IndexOptions=Index vector (dialog)  Indices=[2 1]  OutputSizes=1
  Z : Selector  InputPortWidth=3  IndexOptions=Index vector (dialog)  Indices=3  OutputSizes=1
  dUdlambda : Selector  InputPortWidth=3  IndexOptions=Index vector (dialog)  Indices=3  OutputSizes=1
  dUdlambda/(X^2+Y^2) : Product  Inputs=*/
  dUdphi : Selector  InputPortWidth=3  IndexOptions=Index vector (dialog)  Indices=2  OutputSizes=1
  dUdphi*Z/den : Product  Inputs=**/
  "gx, gy" : Outport  VectorParamsAs1DForOutWhenUnconnected=off
  wires:
  Sum2/1 -> "gx, gy"/1
  X^2+Y^2/1 -> dUdlambda/(X^2+Y^2)/2
  sqrt(X^2+Y^2)/1 -> (r^2)*sqrt()/2
  r^2/1 -> (r^2)*sqrt()/1
  dUdr/r/1 -> Sum/1
  Gain/1 -> Sum2/2
  Xecef/1 -> Y,X/1
  " Xecef"/1 -> "X,Y "/1
  Product1/1 -> Gain/1
  Product/1 -> Sum2/1
  Y,X/1 -> Product1/1
  "X,Y "/1 -> Product/1
  Sum/1 -> Product/2
  dUdlambda/(X^2+Y^2)/1 -> Product1/2
  dUdphi*Z/den/1 -> Sum/2
  "dUdr dUdphi dUdlambda "/1 -> dUdlambda/1, dUdphi/1
  " Xecef "/1 -> Z/1
  dUdphi/1 -> dUdphi*Z/den/1
  Z/1 -> dUdphi*Z/den/2
  (r^2)*sqrt()/1 -> dUdphi*Z/den/3
  dUdlambda/1 -> dUdlambda/(X^2+Y^2)/1

== system aerolibgravity2/Spherical Harmonic Gravity Model/Calculate gravity in ECEF frame/special case - North//South Geographic Pole ==
  Action Port : ActionPort
  zero : Constant  Value=[0 0]
  "gx, gy" : Outport  InitialOutput=[0 0]  VectorParamsAs1DForOutWhenUnconnected=off
  wires:
  zero/1 -> "gx, gy"/1

== system aerolibgravity2/Spherical Harmonic Gravity Model/Get Cosine and Sine of Latitude and Longitude/Test for less than eps ==
  In1 : Inport
  <= eps : simulink/Logic and Bit Operations/Compare To Constant  relop=<=  const=eps  OutDataTypeStr=uint8
  Abs : Abs
  Switch : Switch  Threshold=1
  Zero : Constant  Value=0
  Out1 : Outport  VectorParamsAs1DForOutWhenUnconnected=off
  wires:
  <= eps/1 -> Switch/2
  In1/1 -> Switch/3, Abs/1
  Zero/1 -> Switch/1
  Switch/1 -> Out1/1
  Abs/1 -> <= eps/1

== system aerolibgravity2/Spherical Harmonic Gravity Model/Get Cosine and Sine of Latitude and Longitude/Test for less than eps  ==
  In1 : Inport
  <= eps : simulink/Logic and Bit Operations/Compare To Constant  relop=<=  const=eps  OutDataTypeStr=uint8
  Abs : Abs
  Switch : Switch  Threshold=1
  Zero : Constant  Value=0
  Out1 : Outport  VectorParamsAs1DForOutWhenUnconnected=off
  wires:
  Switch/1 -> Out1/1
  Zero/1 -> Switch/1
  In1/1 -> Switch/3, Abs/1
  <= eps/1 -> Switch/2
  Abs/1 -> <= eps/1

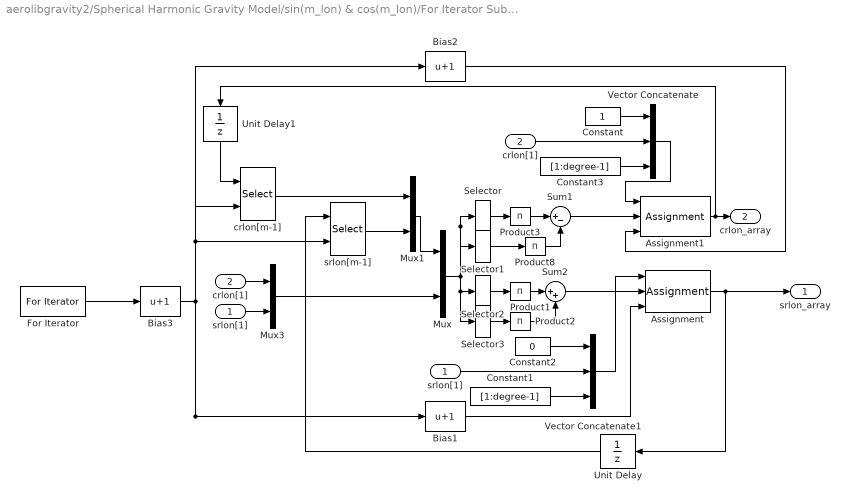
== system aerolibgravity2/Spherical Harmonic Gravity Model/sin(m_lon) & cos(m_lon)/For Iterator Subsystem ==
  srlon[1] : Inport
  crlon[1] : Inport  Port=2
  Assignment : Assignment  IndexMode=Zero-based  DiagnosticForDimensions=Error  IndexOptions=Index vector (port)  Indices=1  OutputSizes=[1 1]
  Assignment1 : Assignment  IndexMode=Zero-based  DiagnosticForDimensions=Error  IndexOptions=Index vector (port)  Indices=1  OutputSizes=[1 1]
  Bias1 : Bias  Bias=1
  Bias2 : Bias  Bias=1
  Bias3 : Bias  Bias=1
  Constant : Constant
  Constant1 : Constant  Value=[1:degree-1]  OutDataTypeStr=Inherit: Inherit via back propagation
  Constant2 : Constant  Value=0
  Constant3 : Constant  Value=[1:degree-1]  OutDataTypeStr=Inherit: Inherit via back propagation
  For Iterator : ForIterator  IterationLimit=degree-1  IndexMode=Zero-based  IterationVariableDataType=double
  Mux : Mux  Inputs=[2 2]
  Mux1 : Mux  Inputs=2
  Mux3 : Mux  Inputs=2
  Product{1..3,8} (4 alike) : Product  Inputs=1  SaturateOnIntegerOverflow=on  OutDataTypeStr=Inherit: Same as first input
  Selector : Selector  IndexMode=Zero-based  InputPortWidth=4  IndexOptions=Index vector (dialog)  Indices=[0 2]  OutputSizes=1
  Selector1 : Selector  IndexMode=Zero-based  InputPortWidth=4  IndexOptions=Index vector (dialog)  Indices=[1 3]  OutputSizes=1
  Selector2 : Selector  IndexMode=Zero-based  InputPortWidth=4  IndexOptions=Index vector (dialog)  Indices=[0 3]  OutputSizes=1
  Selector3 : Selector  IndexMode=Zero-based  InputPortWidth=4  IndexOptions=Index vector (dialog)  Indices=[1 2]  OutputSizes=1
  Sum1 : Sum  Inputs=|+-  SaturateOnIntegerOverflow=on
  Sum2 : Sum  Inputs=|++  SaturateOnIntegerOverflow=on
  Unit Delay : UnitDelay  SampleTime=-1  HasFrameUpgradeWarning=on
  Unit Delay1 : UnitDelay  InitialCondition=1  SampleTime=-1  HasFrameUpgradeWarning=on
  Vector Concatenate : Concatenate  NumInputs=3
  Vector Concatenate1 : Concatenate  NumInputs=3
  "crlon[1] " : InportShadow  Port=2
  crlon[m-1] : Selector  IndexMode=Zero-based  InputPortWidth=degree+1  IndexOptions=Index vector (port)  Indices=[1 3]  OutputSizes=1
  "srlon[1] " : InportShadow
  srlon[m-1] : Selector  IndexMode=Zero-based  InputPortWidth=degree+1  IndexOptions=Index vector (port)  Indices=[1 3]  OutputSizes=1
  srlon_array : Outport  InitialOutput=[0 0 1:(degree-1)]  VectorParamsAs1DForOutWhenUnconnected=off
  crlon_array : Outport  Port=2  InitialOutput=[1 1 1:(degree-1)]  VectorParamsAs1DForOutWhenUnconnected=off
  wires:
  Unit Delay1/1 -> crlon[m-1]/1
  Unit Delay/1 -> srlon[m-1]/1
  Mux1/1 -> Mux/1
  crlon[m-1]/1 -> Mux1/1
  srlon[m-1]/1 -> Mux1/2
  "srlon[1] "/1 -> Vector Concatenate1/2
  Constant1/1 -> Vector Concatenate1/3
  "crlon[1] "/1 -> Vector Concatenate/2
  Constant3/1 -> Vector Concatenate/3
  Vector Concatenate1/1 -> Assignment/1
  Assignment/1 -> Unit Delay/1, srlon_array/1
  Sum1/1 -> Assignment1/2
  Sum2/1 -> Assignment/2
  Product2/1 -> Sum2/2
  Product1/1 -> Sum2/1
  Product8/1 -> Sum1/2
  Product3/1 -> Sum1/1
  Assignment1/1 -> Unit Delay1/1, crlon_array/1
  crlon[1]/1 -> Mux3/1
  srlon[1]/1 -> Mux3/2
  For Iterator/1 -> Bias3/1
  Vector Concatenate/1 -> Assignment1/1
  Selector/1 -> Product3/1
  Mux/1 -> Selector/1, Selector1/1, Selector3/1, Selector2/1
  Selector1/1 -> Product8/1
  Selector2/1 -> Product1/1
  Selector3/1 -> Product2/1
  Mux3/1 -> Mux/2
  Constant/1 -> Vector Concatenate/1
  Constant2/1 -> Vector Concatenate1/1
  Bias2/1 -> Assignment1/3
  Bias1/1 -> Assignment/3
  Bias3/1 -> crlon[m-1]/2, srlon[m-1]/2, Bias1/1, Bias2/1

== system aerolibgravity2/Spherical Harmonic Gravity Model/sin(m_lon) & cos(m_lon)/Test for less than eps ==
  In1 : Inport
  <= eps : simulink/Logic and Bit Operations/Compare To Constant  relop=<=  const=eps  OutDataTypeStr=uint8
  Abs : Abs
  Switch : Switch  Threshold=1
  Zero : Constant  Value=0
  Out1 : Outport  VectorParamsAs1DForOutWhenUnconnected=off
  wires:
  <= eps/1 -> Switch/2
  In1/1 -> Switch/3, Abs/1
  Zero/1 -> Switch/1
  Switch/1 -> Out1/1
  Abs/1 -> <= eps/1

== system aerolibgravity2/Spherical Harmonic Gravity Model/sin(m_lon) & cos(m_lon)/Test for less than eps  ==
  In1 : Inport
  <= eps : simulink/Logic and Bit Operations/Compare To Constant  relop=<=  const=eps  OutDataTypeStr=uint8
  Abs : Abs
  Switch : Switch  Threshold=1
  Zero : Constant  Value=0
  Out1 : Outport  VectorParamsAs1DForOutWhenUnconnected=off
  wires:
  Switch/1 -> Out1/1
  Zero/1 -> Switch/1
  In1/1 -> Switch/3, Abs/1
  <= eps/1 -> Switch/2
  Abs/1 -> <= eps/1

== system aerolibgravity2/Zonal Harmonic Gravity Model/Calculate gravity in ECEF frame/gx & gy ==
  Xecef : Inport
  g_trans : Inport  Port=2
  r : Inport  Port=3
  g_radial/r : Inport  Port=4
  Compare To Zero : simulink/Logic and Bit Operations/Compare To Zero  relop===  OutDataTypeStr=boolean  ZeroCross=off
  Constant : Constant
  Logical Operator : Logic  Inputs=1  AllPortsSameDT=off  OutDataTypeStr=boolean
  Product : Product  RndMeth=Zero
  Product1 : Product  Inputs=*//*  RndMeth=Zero
  Product2 : Product  RndMeth=Zero
  Product3 : Product  RndMeth=Zero
  "Selector x " : Selector  InputPortWidth=3  IndexOptions=Index vector (dialog)  Indices=1  OutputSizes=1
  Selector x & y : Selector  InputPortWidth=3  IndexOptions=Index vector (dialog)  Indices=[1 2]  OutputSizes=1
  Selector y : Selector  InputPortWidth=3  IndexOptions=Index vector (dialog)  Indices=2  OutputSizes=1
  Selector z : Selector  InputPortWidth=3  IndexOptions=Index vector (dialog)  Indices=3  OutputSizes=1
  Special case for polar : Switch  Criteria=u2 ~= 0
  Sum : Sum  Inputs=|+-
  Sum of Elements : Sum  Inputs=+
  sqrt : Sqrt  AlgorithmType=Newton-Raphson  SaturateOnIntegerOverflow=on
  gx : Outport  VectorParamsAs1DForOutWhenUnconnected=off
  gy : Outport  Port=2  VectorParamsAs1DForOutWhenUnconnected=off
  wires:
  Constant/1 -> Special case for polar/1
  Special case for polar/1 -> Product1/2
  Logical Operator/1 -> Special case for polar/2
  Compare To Zero/1 -> Logical Operator/1
  Sum of Elements/1 -> sqrt/1
  Product/1 -> Sum of Elements/1
  Selector x & y/1 -> Compare To Zero/1, Product/2, Product/1
  Selector y/1 -> Product3/2
  Product3/1 -> gy/1
  "Selector x "/1 -> Product2/1
  Sum/1 -> Product3/1, Product2/2
  Product2/1 -> gx/1
  g_trans/1 -> Product1/4
  Product1/1 -> Sum/2
  r/1 -> Product1/3
  sqrt/1 -> Special case for polar/3
  Selector z/1 -> Product1/1
  g_radial/r/1 -> Sum/1
  Xecef/1 -> Selector x & y/1, Selector y/1, Selector z/1, "Selector x "/1

== system aerolibgravity2/Zonal Harmonic Gravity Model/Calculate gravity in ECEF frame/gz ==
  g_radial/r : Inport
  r : Inport  Port=2
  g_trans : Inport  Port=3
  Xecef : Inport  Port=4
  Product : Product  RndMeth=Zero
  Product1 : Product  Inputs=*/*  RndMeth=Zero
  Product2 : Product  RndMeth=Zero
  Selector x & y : Selector  InputPortWidth=3  IndexOptions=Index vector (dialog)  Indices=[1 2]  OutputSizes=1
  Selector z : Selector  InputPortWidth=3  IndexOptions=Index vector (dialog)  Indices=3  OutputSizes=1
  Sum : Sum  Inputs=|++
  Sum of Elements : Sum  Inputs=+
  sqrt : Sqrt  AlgorithmType=Newton-Raphson  SaturateOnIntegerOverflow=on
  gz : Outport  VectorParamsAs1DForOutWhenUnconnected=off
  wires:
  Sum of Elements/1 -> sqrt/1
  Product2/1 -> Sum of Elements/1
  Selector x & y/1 -> Product2/1, Product2/2
  Sum/1 -> gz/1
  Product1/1 -> Sum/2
  g_trans/1 -> Product1/3
  r/1 -> Product1/2
  sqrt/1 -> Product1/1
  Xecef/1 -> Selector x & y/1, Selector z/1
  Product/1 -> Sum/1
  Selector z/1 -> Product/2
  g_radial/r/1 -> Product/1

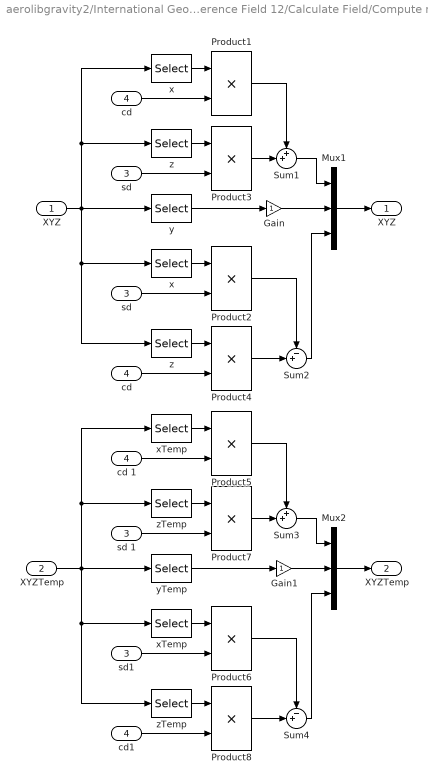
== system aerolibgravity2/International Geomagnetic Reference Field 12/Calculate Field/Compute magnetic vector in spherical coordinates/Calculate X, Z, XTemp and ZTemp ==
  "XYZ " : Inport
  "XYZTemp " : Inport  Port=2
  sd : Inport  Port=3
  cd : Inport  Port=4
  Gain : Gain
  Gain1 : Gain
  Mux1 : Mux  Inputs=3
  Mux2 : Mux  Inputs=3
  Product{1..8} (8 alike) : Product  SaturateOnIntegerOverflow=on  OutDataTypeStr=Inherit: Same as first input
  Sum1 : Sum  Inputs=++|  SaturateOnIntegerOverflow=on
  Sum2 : Sum  Inputs=-+|  SaturateOnIntegerOverflow=on
  Sum3 : Sum  Inputs=++|  SaturateOnIntegerOverflow=on
  Sum4 : Sum  Inputs=-+|  SaturateOnIntegerOverflow=on
  "cd " : InportShadow  Port=4
  cd 1 : InportShadow  Port=4
  cd1 : InportShadow  Port=4
  "sd " : InportShadow  Port=3
  sd 1 : InportShadow  Port=3
  sd1 : InportShadow  Port=3
  x : Selector  InputPortWidth=3  IndexOptions=Index vector (dialog)  Indices=1  OutputSizes=1
  "x " : Selector  InputPortWidth=3  IndexOptions=Index vector (dialog)  Indices=1  OutputSizes=1
  xTemp : Selector  InputPortWidth=3  IndexOptions=Index vector (dialog)  Indices=1  OutputSizes=1
  "xTemp " : Selector  InputPortWidth=3  IndexOptions=Index vector (dialog)  Indices=1  OutputSizes=1
  y : Selector  InputPortWidth=3  IndexOptions=Index vector (dialog)  Indices=2  OutputSizes=1
  yTemp : Selector  InputPortWidth=3  IndexOptions=Index vector (dialog)  Indices=2  OutputSizes=1
  z : Selector  InputPortWidth=3  IndexOptions=Index vector (dialog)  Indices=3  OutputSizes=1
  "z " : Selector  InputPortWidth=3  IndexOptions=Index vector (dialog)  Indices=3  OutputSizes=1
  zTemp : Selector  InputPortWidth=3  IndexOptions=Index vector (dialog)  Indices=3  OutputSizes=1
  "zTemp " : Selector  InputPortWidth=3  IndexOptions=Index vector (dialog)  Indices=3  OutputSizes=1
  XYZ : Outport  VectorParamsAs1DForOutWhenUnconnected=off
  XYZTemp : Outport  Port=2  VectorParamsAs1DForOutWhenUnconnected=off
  wires:
  Mux1/1 -> XYZ/1
  "XYZ "/1 -> y/1, "x "/1, "z "/1, z/1, x/1
  y/1 -> Gain/1
  x/1 -> Product1/1
  cd/1 -> Product1/2
  "x "/1 -> Product2/1
  sd/1 -> Product2/2
  z/1 -> Product3/1
  "sd "/1 -> Product3/2
  "z "/1 -> Product4/1
  "cd "/1 -> Product4/2
  Product3/1 -> Sum1/2
  Product1/1 -> Sum1/1
  Sum1/1 -> Mux1/1
  Product4/1 -> Sum2/2
  Product2/1 -> Sum2/1
  Sum2/1 -> Mux1/3
  Mux2/1 -> XYZTemp/1
  "XYZTemp "/1 -> xTemp/1, zTemp/1, "zTemp "/1, "xTemp "/1, yTemp/1
  yTemp/1 -> Gain1/1
  xTemp/1 -> Product5/1
  cd 1/1 -> Product5/2
  "xTemp "/1 -> Product6/1
  sd1/1 -> Product6/2
  zTemp/1 -> Product7/1
  sd 1/1 -> Product7/2
  "zTemp "/1 -> Product8/1
  cd1/1 -> Product8/2
  Product7/1 -> Sum3/2
  Product5/1 -> Sum3/1
  Sum3/1 -> Mux2/1
  Product8/1 -> Sum4/2
  Product6/1 -> Sum4/1
  Sum4/1 -> Mux2/3
  Gain/1 -> Mux1/2
  Gain1/1 -> Mux2/2
